simulink model "T1"  (R2015a)
settings: Solver=ode45  StartTime=0.0  StopTime=10.0  RelTol=1e-3
settings Model: Creator=Benjamin Nicolas  LastModifiedBy=Benjamin Nicolas

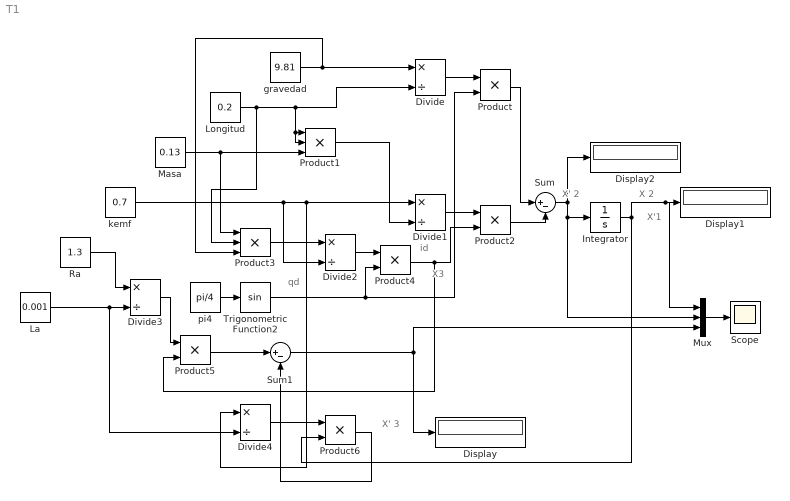
== system T1 ==
  note: X'1
  note: X' 3
  note: id
  note: qd
  note: X 2
  note: X' 2
  note: X3
  Display : Display
  Display1 : Display
  Display2 : Display
  Divide{,1..4} (5 alike) : Product  Inputs=*/  SaturateOnIntegerOverflow=on  RndMeth=Zero
  Integrator : Integrator  InitialCondition=1
  La : Constant  Value=0.001
  "Longitud " : Constant  Value=0.2
  Masa : Constant  Value=0.13
  Mux : Mux  Inputs=3
  Product{,2,4..6} (5 alike) : Product
  Product1 : Product  Inputs=3
  Product3 : Product  Inputs=3
  Ra : Constant  Value=1.3
  Scope : Scope
  Sum : Sum  Inputs=|+-
  Sum1 : Sum  Inputs=|+-
  Trigonometric Function2 : Trigonometry
  gravedad : Constant  Value=9.81
  "kemf " : Constant  Value=0.7
  "pi4 " : Constant  Value=pi/4
  wires:
  gravedad/1 -> Product3/3, Divide/1
  "Longitud "/1 -> Product3/2, Product1/2, Product1/1, Divide/2
  Divide/1 -> Product/1
  Product/1 -> Sum/1
  "kemf "/1 -> Divide2/2, Divide4/1, Divide1/1
  Product1/1 -> Divide1/2
  Masa/1 -> Product3/1, Product1/3
  Divide1/1 -> Product2/1
  Product2/1 -> Sum/2
  Product3/1 -> Divide2/1
  Trigonometric Function2/1 -> Product4/2, Product/2
  "pi4 "/1 -> Trigonometric Function2/1
  Sum/1 -> Integrator/1, Mux/2, Display2/1
  Ra/1 -> Divide3/1
  La/1 -> Divide4/2, Divide3/2
  Divide2/1 -> Product4/1
  Product4/1 -> Product5/2, Product2/2
  Divide3/1 -> Product5/1
  Integrator/1 -> Mux/1, Display1/1, Product6/2
  Product5/1 -> Sum1/1
  Divide4/1 -> Product6/1
  Product6/1 -> Sum1/2
  Sum1/1 -> Display/1, Mux/3
  Mux/1 -> Scope/1
